simulink model "motor_control_velocity"  (R2019b)
settings: Solver=VariableStepAuto  StartTime=0.0  StopTime=0.1  RelTol=1e-3
undefined symbols (not defined in the file): Bnew, Gear_Ratio, Jnew, Ke, Ki_current, Ki_velocity, Kp_current, Kp_velocity, Kt, La, Ra, V
libraries: simulink_extras x1
settings Model: Creator=이종수  LastModifiedBy=이종수

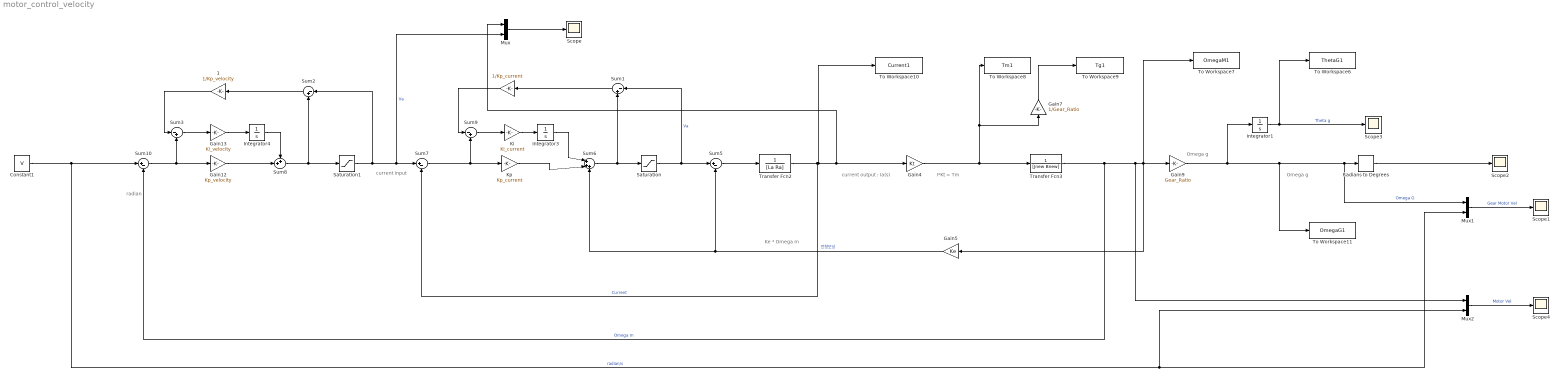
== system motor_control_velocity ==
  note: radian
  note: current input
  note: I*Kt = Tm
  note: current output : Ia(s)
  note: Ke * Omega m
  note: Omega g
  note: Omega g
  " " : Gain  Gain=1/Kp_current
  " 1" : Gain  Gain=1/Kp_velocity
  Constant1 : Constant  Value=V
  Gain12 : Gain  Gain=Kp_velocity
  Gain13 : Gain  Gain=Ki_velocity
  Gain4 : Gain  Gain=Kt
  Gain5 : Gain  Gain=Ke
  Gain7 : Gain  Gain=1/Gear_Ratio
  Gain9 : Gain  Gain=Gear_Ratio
  Integrator1 : Integrator
  Integrator3 : Integrator
  Integrator4 : Integrator
  "Ki " : Gain  Gain=Ki_current
  "Kp " : Gain  Gain=Kp_current
  Mux : Mux  Inputs=2
  Mux1 : Mux  Inputs=2
  Mux2 : Mux  Inputs=2
  Radians to Degrees : simulink_extras/Transformations/Radians to Degrees
  Saturation : Saturate
  Saturation1 : Saturate
  Scope{,1..4} (5 alike) : Scope
  Sum{1..3,9} (4 alike) : Sum  Inputs=|-+
  Sum10 : Sum  Inputs=|+-
  Sum5 : Sum  Inputs=|+-
  Sum6 : Sum  Inputs=|+++
  Sum7 : Sum  Inputs=|+-
  Sum8 : Sum  Inputs=++|
  To Workspace10 : ToWorkspace  VariableName=Current1  SaveFormat=Structure With Time  SampleTime=-1
  To Workspace11 : ToWorkspace  VariableName=OmegaG1  SaveFormat=Structure With Time  SampleTime=-1
  To Workspace6 : ToWorkspace  VariableName=ThetaG1  SaveFormat=Structure With Time  SampleTime=-1
  To Workspace7 : ToWorkspace  VariableName=OmegaM1  SaveFormat=Structure With Time  SampleTime=-1
  To Workspace8 : ToWorkspace  VariableName=Tm1  SaveFormat=Structure With Time  SampleTime=-1
  To Workspace9 : ToWorkspace  VariableName=Tg1  SaveFormat=Structure With Time  SampleTime=-1
  Transfer Fcn2 : TransferFcn  Denominator=[La Ra]
  Transfer Fcn3 : TransferFcn  Denominator=[Jnew Bnew]
  wires:
  Transfer Fcn3/1 -> Mux2/1, To Workspace7/1, Gain5/1, Gain9/1, Sum10/2  "Omega m"
  Gain9/1 -> Mux1/1, Radians to Degrees/1, To Workspace11/1, Integrator1/1  "Omega G"
  Gain7/1 -> To Workspace9/1
  Gain5/1 -> Sum6/3, Sum5/2  "전향보상"
  Gain4/1 -> Transfer Fcn3/1, Gain7/1, To Workspace8/1
  Integrator1/1 -> To Workspace6/1, Scope3/1  "Theta g"
  Transfer Fcn2/1 -> Mux/1, Gain4/1, To Workspace10/1, Sum7/2  "Current"
  "Ki "/1 -> Integrator3/1
  Sum7/1 -> "Kp "/1, Sum9/2
  Sum5/1 -> Transfer Fcn2/1
  Gain13/1 -> Integrator4/1
  Sum6/1 -> Sum1/2, Saturation/1
  Saturation/1 -> Sum1/1, Sum5/1  "Va"
  Sum1/1 -> " "/1
  Sum9/1 -> "Ki "/1
  " "/1 -> Sum9/1
  "Kp "/1 -> Sum6/2
  Integrator3/1 -> Sum6/1
  Gain12/1 -> Sum8/2
  Integrator4/1 -> Sum8/1
  Sum10/1 -> Sum3/2, Gain12/1
  Sum8/1 -> Saturation1/1, Sum2/2
  Constant1/1 -> Mux2/2, Mux1/2, Sum10/1  "radian/s"
  Radians to Degrees/1 -> Scope2/1
  Mux1/1 -> Scope1/1  "Gear Motor Vel"
  Mux2/1 -> Scope4/1  "Motor Vel"
  Mux/1 -> Scope/1
  Saturation1/1 -> Sum2/1, Mux/2, Sum7/1  "Va"
  Sum2/1 -> " 1"/1
  Sum3/1 -> Gain13/1
  " 1"/1 -> Sum3/1
